simulink model "Controlador_pitch"  (R2022a)
settings: Solver=VariableStepAuto  StartTime=0.0  StopTime=5  RelTol=1e-3
undefined symbols (not defined in the file): pitch_ref
settings Model: Creator=juani  LastModifiedBy=juani
settings SolverCC: ZeroCrossAlgorithm=Adaptive
settings DebuggingCC: IgnoredZcDiagnostic=none

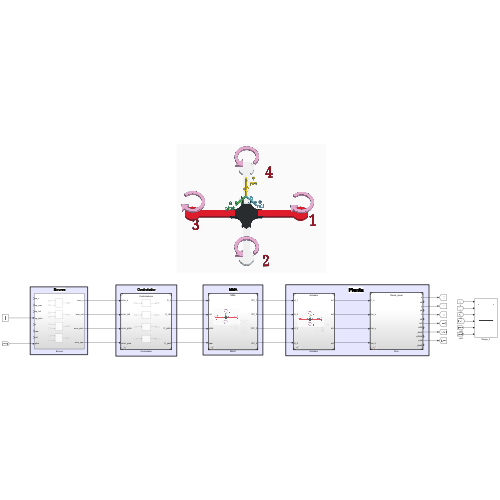
[thumbnail: Simulink's stored preview of the top-level diagram]
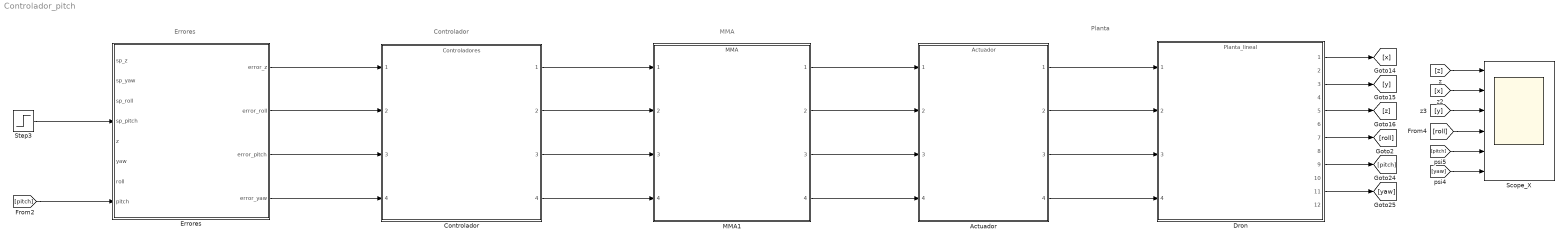
== system Controlador_pitch ==
  note: Errores
  note: MMA
  note: Planta
  note: Controlador
  Actuador : ModelReference  ModelNameDialog=Actuador.slx  SimulationMode=Normal  ModelReferenceVersion=1.14
  Controlador : ModelReference  ModelNameDialog=Controladores.slx  SimulationMode=Normal  ModelReferenceVersion=1.14
  Dron : ModelReference  ModelNameDialog=Planta_lineal.slx  SimulationMode=Normal  ModelReferenceVersion=1.4
  Errores : Subsystem
  MMA1 : ModelReference  ModelNameDialog=MMA.slx  SimulationMode=Normal  ModelReferenceVersion=1.28
  Scope_X : Scope  NumInputPorts=6
  Step3 : Step  Time=0.2  After=pitch_ref  SampleTime=0
  wires:
  Errores/3(error_pitch) -> Controlador/3
  MMA1/3 -> Actuador/3
  [roll] -> Scope_X/4
  [pitch] -> Scope_X/5
  MMA1/2 -> Actuador/2
  Actuador/2 -> Dron/2
  Dron/1 -> [x]
  MMA1/1 -> Actuador/1
  MMA1/4 -> Actuador/4
  Controlador/4 -> MMA1/4
  [yaw] -> Scope_X/6
  Controlador/1 -> MMA1/1
  [y] -> Scope_X/3
  Dron/7 -> [roll]
  [z] -> Scope_X/1
  Dron/3 -> [y]
  Errores/2(error_roll) -> Controlador/2
  Actuador/1 -> Dron/1
  Errores/4(error_yaw) -> Controlador/4
  Controlador/3 -> MMA1/3
  Errores/1(error_z) -> Controlador/1
  Dron/11 -> [yaw]
  Actuador/3 -> Dron/3
  Controlador/2 -> MMA1/2
  [x] -> Scope_X/2
  Actuador/4 -> Dron/4
  Dron/5 -> [z]
  Dron/9 -> [pitch]
  Step3/1 -> Errores/4(sp_pitch)
  [pitch] -> Errores/8(pitch)

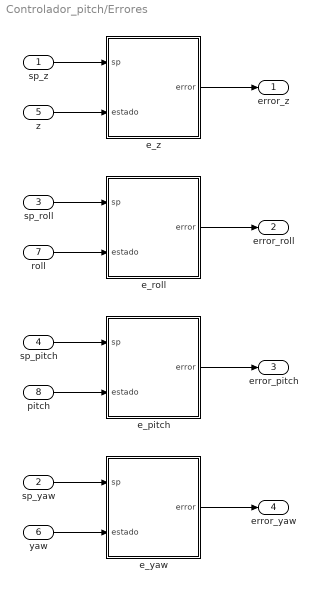
== system Controlador_pitch/Errores ==
  sp_z : Inport
  sp_yaw : Inport  Port=2
  sp_roll : Inport  Port=3
  sp_pitch : Inport  Port=4
  z : Inport  Port=5
  yaw : Inport  Port=6
  roll : Inport  Port=7
  pitch : Inport  Port=8
  e_pitch : Subsystem
  e_roll : Subsystem
  e_yaw : Subsystem
  e_z : Subsystem
  error_z : Outport
  error_roll : Outport  Port=2
  error_pitch : Outport  Port=3
  error_yaw : Outport  Port=4
  wires:
  sp_z/1 -> e_z/1(sp)
  sp_yaw/1 -> e_yaw/1(sp)
  sp_pitch/1 -> e_pitch/1(sp)
  sp_roll/1 -> e_roll/1(sp)
  z/1 -> e_z/2(estado)
  yaw/1 -> e_yaw/2(estado)
  roll/1 -> e_roll/2(estado)
  pitch/1 -> e_pitch/2(estado)
  e_z/1(error) -> error_z/1
  e_yaw/1(error) -> error_yaw/1
  e_pitch/1(error) -> error_pitch/1
  e_roll/1(error) -> error_roll/1

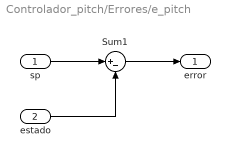
== system Controlador_pitch/Errores/e_pitch ==
  sp : Inport
  estado : Inport  Port=2
  Sum1 : Sum  Inputs=|+-
  error : Outport
  wires:
  sp/1 -> Sum1/1
  Sum1/1 -> error/1
  estado/1 -> Sum1/2

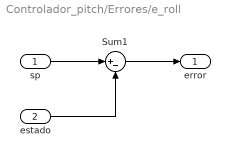
== system Controlador_pitch/Errores/e_roll ==
  sp : Inport
  estado : Inport  Port=2
  Sum1 : Sum  Inputs=|+-
  error : Outport
  wires:
  sp/1 -> Sum1/1
  Sum1/1 -> error/1
  estado/1 -> Sum1/2

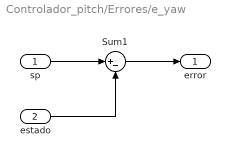
== system Controlador_pitch/Errores/e_yaw ==
  sp : Inport
  estado : Inport  Port=2
  Sum1 : Sum  Inputs=|+-
  error : Outport
  wires:
  sp/1 -> Sum1/1
  Sum1/1 -> error/1
  estado/1 -> Sum1/2

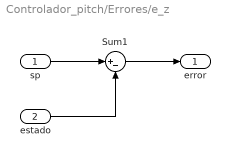
== system Controlador_pitch/Errores/e_z ==
  sp : Inport
  estado : Inport  Port=2
  Sum1 : Sum  Inputs=|+-
  error : Outport
  wires:
  sp/1 -> Sum1/1
  Sum1/1 -> error/1
  estado/1 -> Sum1/2
